simulink model "quadrotor_demo"  (Simulink 7.6)
settings: Solver=ode45  StartTime=0.0  StopTime=100  RelTol=1e-3
undefined symbols (not defined in the file): STARMAC, uav_utilities
libraries: simulink x9, aero_sim_lib x8
(part 1 of 2)
settings Model: Creator=Administrator  LastModifiedBy=jporter  SimulationMode=rapid-accelerator
settings OptimizationCC: InitFltsAndDblsToZero=on
settings DebuggingCC: SignalRangeChecking=warning  ParameterDowncastMsg=warning  ParameterOverflowMsg=warning
settings HardwareCC: ProdLargestAtomicInteger=Long  ProdLargestAtomicFloat=Float  ProdEndianess=LittleEndian  ProdHWDeviceType=ARM Compatible->ARM 7
settings SFSimCC: SimParseCustomCode=off

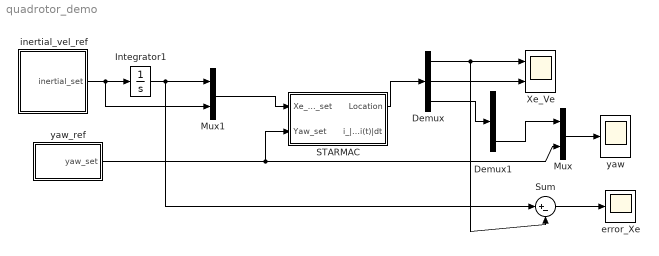
== system quadrotor_demo ==
  Demux : Demux  Outputs=[3,3,3]
  Demux1 : Demux  Outputs=3
  Integrator1 : Integrator
  Mux : Mux  Inputs=2
  Mux1 : Mux  Inputs=2
  STARMAC : Subsystem  AncestorBlock=uav_utilities/STARMAC  MinMaxOverflowLogging=MinMaxAndOverflow
  Sum : Sum  Inputs=|+-
  Xe_Ve : Scope  NumInputPorts=2
      settings: YMin=-500~-10  YMax=6500~110  SampleInput=on  SampleTime=100/5000
  error_Xe : Scope
      settings: YMin=-50  YMax=60  SaveName=error_data  Decimation=10  SampleInput=on  SampleTime=100/5000
  inertial_vel_ref : Subsystem
  yaw : Scope
      settings: YMin=-1  YMax=1  SaveName=ScopeData2  SampleInput=on  SampleTime=100/5000
  yaw_ref : Subsystem
  wires:
  inertial_vel_ref/1(inertial_set) -> Integrator1/1, Mux1/2
  yaw_ref/1(yaw_set) -> STARMAC/2(Yaw_set), Mux/2
  Sum/1 -> error_Xe/1
  STARMAC/1(Location) -> Demux/1
  Demux/1 -> Sum/2, Xe_Ve/1
  Demux/2 -> Xe_Ve/2
  Mux/1 -> yaw/1
  Demux/3 -> Demux1/1
  Demux1/3 -> Mux/1
  Integrator1/1 -> Mux1/1, Sum/1
  Mux1/1 -> STARMAC/1(Xe_Ve_set)

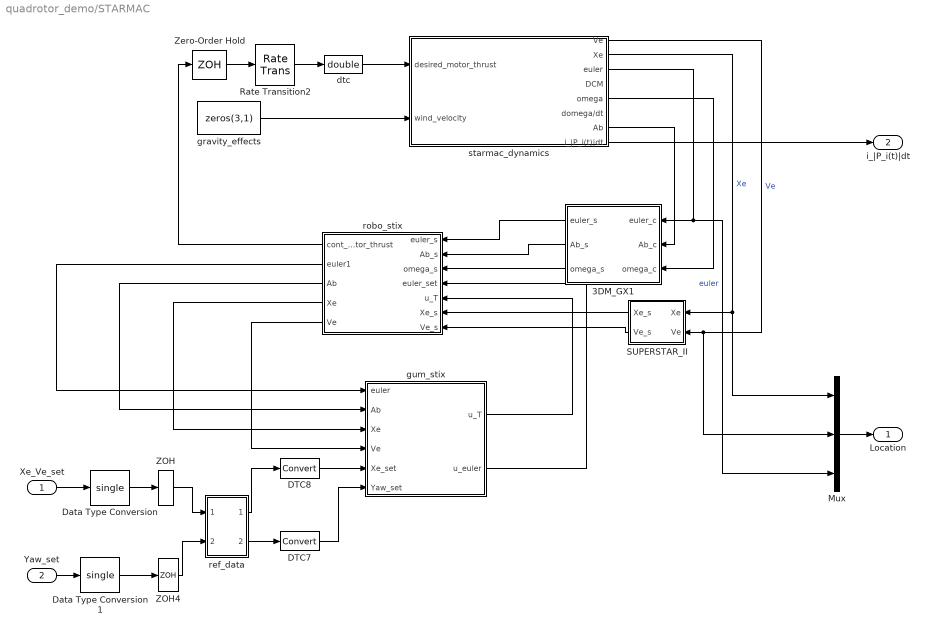
== system quadrotor_demo/STARMAC ==
  Xe_Ve_set : Inport  PortDimensions=[6]
  Yaw_set : Inport  Port=2  PortDimensions=[1]
  3DM_GX1 : Subsystem  mask{a_g_s=7000, g_max=5, g_g_s=8500, omega_max=300, Ts=.02}
      mask prompts: a_g_s "AccelGainScale:"; g_max "Max G (1 G = 9.81 m/s^2):"; g_g_s "GyroGainScale:"; omega_max "Mav Angular Velocity (deg/sec):"; Ts "Sample Rate (seconds):"
  DTC7 : DataTypeConversion
  DTC8 : DataTypeConversion
  Data Type Conversion : DataTypeConversion  OutDataTypeStr=single
  Data Type Conversion1 : DataTypeConversion  OutDataTypeStr=single
  Mux : Mux  Inputs=[3 3 3]
  Rate Transition2 : RateTransition
  SUPERSTAR_II : Subsystem  mask{Ts=.2}
      mask prompts: Ts "Sample Rate (seconds):"
  ZOH : ZeroOrderHold  SampleTime=.02
  ZOH4 : ZeroOrderHold  SampleTime=.02
  Zero-Order Hold : ZeroOrderHold  SampleTime=.02
  dtc : DataTypeConversion  OutDataTypeStr=double
  gravity_effects : Constant  Value=zeros(3,1)  OutDataTypeStr=double
  gum_stix : Subsystem
  ref_data : Subsystem
  robo_stix : Subsystem
  starmac_dynamics : Subsystem  AncestorBlock=aero_sim_lib/starmac_dynamics
  Location : Outport
  i_|P_i(t)|dt : Outport  Port=2
  wires:
  starmac_dynamics/8(i_|P_i(t)|dt) -> i_|P_i(t)|dt/1
  ref_data/2(Out2) -> DTC7/1
  Yaw_set/1 -> Data Type Conversion1/1
  Xe_Ve_set/1 -> Data Type Conversion/1
  Mux/1 -> Location/1
  robo_stix/1(cont_motor_thrust) -> Zero-Order Hold/1
  starmac_dynamics/3(euler) -> 3DM_GX1/1(euler_c), Mux/3  "euler"
  starmac_dynamics/7(Ab) -> 3DM_GX1/2(Ab_c)
  3DM_GX1/1(euler_s) -> robo_stix/1(euler_s)
  3DM_GX1/2(Ab_s) -> robo_stix/2(Ab_s)
  3DM_GX1/3(omega_s) -> robo_stix/3(omega_s)
  robo_stix/2(euler1) -> gum_stix/1(euler)
  SUPERSTAR_II/1(Xe_s) -> robo_stix/6(Xe_s)
  SUPERSTAR_II/2(Ve_s) -> robo_stix/7(Ve_s)
  starmac_dynamics/2(Xe) -> SUPERSTAR_II/1(Xe), Mux/1  "Xe"
  starmac_dynamics/1(Ve) -> SUPERSTAR_II/2(Ve), Mux/2  "Ve"
  gravity_effects/1 -> starmac_dynamics/2(wind_velocity)
  gum_stix/1(u_T) -> robo_stix/5(u_T)
  gum_stix/2(u_euler) -> robo_stix/4(euler_set)
  ref_data/1(Out1) -> DTC8/1
  dtc/1 -> starmac_dynamics/1(desired_motor_thrust)
  starmac_dynamics/5(omega) -> 3DM_GX1/3(omega_c)
  Zero-Order Hold/1 -> Rate Transition2/1
  Rate Transition2/1 -> dtc/1
  robo_stix/3(Ab) -> gum_stix/2(Ab)
  robo_stix/5(Ve) -> gum_stix/4(Ve)
  ZOH/1 -> ref_data/1(Xe_Ve_set)
  ZOH4/1 -> ref_data/2(yaw_set)
  Data Type Conversion/1 -> ZOH/1
  Data Type Conversion1/1 -> ZOH4/1
  DTC7/1 -> gum_stix/6(Yaw_set)
  DTC8/1 -> gum_stix/5(Xe_set)
  robo_stix/4(Xe) -> gum_stix/3(Xe)

== system quadrotor_demo/inertial_vel_ref ==
  Signal Generator : SignalGenerator  Amplitude=10*[1 -1 -.5]  Frequency=.1*.0625*ones(3,1)
  inertial_set : Outport
  wires:
  Signal Generator/1 -> inertial_set/1

== system quadrotor_demo/yaw_ref ==
  Signal Generator : SignalGenerator  Frequency=2*.0625*0.25
  yaw_set : Outport
  wires:
  Signal Generator/1 -> yaw_set/1

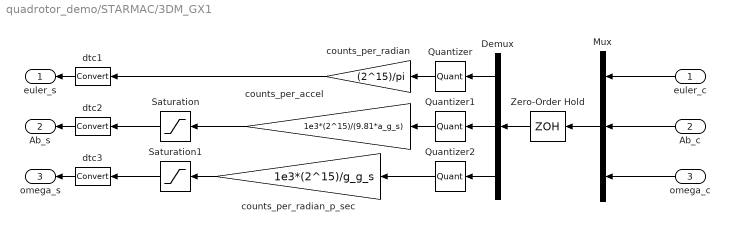
== system quadrotor_demo/STARMAC/3DM_GX1 ==
  euler_c : Inport
  Ab_c : Inport  Port=2
  omega_c : Inport  Port=3
  Demux : Demux  Outputs=[3 3 3]
  Mux : Mux  Inputs=[3 3 3]
  Quantizer : Quantizer  QuantizationInterval=pi/(2^15)*ones(3,1)
  Quantizer1 : Quantizer  QuantizationInterval=g_max*9.81/(2^15)*ones(3,1)
  Quantizer2 : Quantizer  QuantizationInterval=(pi*omega_max/180)/(2^15)*ones(3,1)
  Saturation : Saturate  UpperLimit=((2^15)-1)*ones(3,1)  LowerLimit=-(2^15)*ones(3,1)
  Saturation1 : Saturate  UpperLimit=((2^15)-1)*ones(3,1)  LowerLimit=-(2^15)*ones(3,1)
  Zero-Order Hold : ZeroOrderHold  SampleTime=Ts
  counts_per_accel : Gain  Gain=1e3*(2^15)/(9.81*a_g_s)  OutDataTypeStr=single
  counts_per_radian : Gain  Gain=(2^15)/pi  OutDataTypeStr=single
  counts_per_radian_p_sec : Gain  Gain=1e3*(2^15)/g_g_s  OutDataTypeStr=single
  dtc1 : DataTypeConversion
  dtc2 : DataTypeConversion
  dtc3 : DataTypeConversion
  euler_s : Outport
  Ab_s : Outport  Port=2
  omega_s : Outport  Port=3
  wires:
  Mux/1 -> Zero-Order Hold/1
  euler_c/1 -> Mux/1
  Ab_c/1 -> Mux/2
  omega_c/1 -> Mux/3
  Zero-Order Hold/1 -> Demux/1
  Demux/1 -> Quantizer/1
  Demux/2 -> Quantizer1/1
  Quantizer/1 -> counts_per_radian/1
  Quantizer1/1 -> counts_per_accel/1
  counts_per_accel/1 -> Saturation/1
  Demux/3 -> Quantizer2/1
  counts_per_radian_p_sec/1 -> Saturation1/1
  Quantizer2/1 -> counts_per_radian_p_sec/1
  Saturation/1 -> dtc2/1
  Saturation1/1 -> dtc3/1
  dtc1/1 -> euler_s/1
  dtc2/1 -> Ab_s/1
  dtc3/1 -> omega_s/1
  counts_per_radian/1 -> dtc1/1

== system quadrotor_demo/STARMAC/SUPERSTAR_II ==
  Xe : Inport
  Ve : Inport  Port=2
  Demux : Demux  Outputs=[3 3]
  Mux : Mux  Inputs=[3 3]
  Rate Transition : RateTransition
  ZOH : ZeroOrderHold  SampleTime=Ts
  dtc1 : DataTypeConversion
  dtc2 : DataTypeConversion
  Xe_s : Outport
  Ve_s : Outport  Port=2
  wires:
  ZOH/1 -> Rate Transition/1
  Ve/1 -> Mux/2
  Xe/1 -> Mux/1
  Mux/1 -> ZOH/1
  Demux/1 -> dtc1/1
  Demux/2 -> dtc2/1
  dtc1/1 -> Xe_s/1
  dtc2/1 -> Ve_s/1
  Rate Transition/1 -> Demux/1

== system quadrotor_demo/STARMAC/gum_stix ==
  euler : Inport  OutMin=-pi  OutMax=pi  OutDataTypeStr=fixdt(1,32,28)  PortDimensions=[3]
  Ab : Inport  Port=2  OutMin=-200  OutMax=200  OutDataTypeStr=fixdt(1,32,23)  PortDimensions=[3]
  Xe : Inport  Port=3  OutMin=-2000  OutMax=2000  OutDataTypeStr=fixdt(1,32,20)  PortDimensions=[3]
  Ve : Inport  Port=4  OutMin=-200  OutMax=200  OutDataTypeStr=fixdt(1,32,23)  PortDimensions=[3]
  Xe_set : Inport  Port=5  OutMin=-2000  OutMax=2000  OutDataTypeStr=fixdt(1,32,20)  PortDimensions=[3]
  Yaw_set : Inport  Port=6  OutMin=-pi  OutMax=pi  OutDataTypeStr=fixdt(1,32,29)  PortDimensions=[1]
  DTC : DataTypeConversion
  Demux : Demux  Outputs=3
  body_to_inertial : Subsystem
  inertial_pos_controller : Subsystem
  rate_limiter : Subsystem  mask{wn=2*pi, zeta=0.9, Vmax=2, T=0.02, Hzn1=0, Hzd1=0}
      mask prompts: wn "omega_n"; Vmax "Max velocity"; T "Sample time"; Hzn1 "Filter numerator"; Hzd1 "Filter denominator"
      mask init:
      | Hs=tf([wn^2],[1,2*zeta*wn,wn^2]);
      | Hz=ipesh_transform(Hs,T);
      | Hzn1 = Hz.num{1};
      | %Hzn1 = [0.002488 0.009405 0.002222];
      | Hzd1 = Hz.den{1};
      | %Hzd1 = [1.0000 -1.7834 0.7976];
  sensor_fusion : Subsystem
  u_T : Outport  OutMin=0  OutMax=100  PortDimensions=[1]
  u_euler : Outport  Port=2  OutMin=-pi  OutMax=pi  PortDimensions=[3]
  wires:
  Xe_set/1 -> rate_limiter/1(Xe_set)
  inertial_pos_controller/1(u_T) -> u_T/1
  inertial_pos_controller/2(u_euler) -> u_euler/1
  euler/1 -> body_to_inertial/1(euler), Demux/1
  Ab/1 -> DTC/1
  sensor_fusion/1(Xe) -> inertial_pos_controller/2(Xe)
  sensor_fusion/2(Ve) -> inertial_pos_controller/3(Ve)
  body_to_inertial/1(Xe) -> sensor_fusion/1(Xe_f)
  body_to_inertial/2(Ve) -> sensor_fusion/2(Ve_f)
  Xe/1 -> sensor_fusion/3(Xe_s)
  Ve/1 -> sensor_fusion/4(Ve_s)
  rate_limiter/1(Xr_set) -> inertial_pos_controller/1(Xe_set)
  Demux/3 -> inertial_pos_controller/4(Yaw_actual)
  Yaw_set/1 -> inertial_pos_controller/5(Yaw_set)
  DTC/1 -> body_to_inertial/2(Ab)

== system quadrotor_demo/STARMAC/ref_data ==
  Xe_Ve_set : Inport  PortDimensions=[6]
  yaw_set : Inport  Port=2  PortDimensions=[1]
  Data Type Conversion : DataTypeConversion
  Data Type Conversion1 : DataTypeConversion
  Demux : Demux  Outputs=[3,3]
  Terminator : Terminator
  Out1 : Outport
  Out2 : Outport  Port=2
  wires:
  Demux/2 -> Terminator/1
  Demux/1 -> Data Type Conversion/1
  Data Type Conversion/1 -> Out1/1
  Xe_Ve_set/1 -> Demux/1
  Data Type Conversion1/1 -> Out2/1
  yaw_set/1 -> Data Type Conversion1/1

== system quadrotor_demo/STARMAC/robo_stix ==
  euler_s : Inport  OutMin=-(2^15)  OutMax=2^15  OutDataTypeStr=fixdt(1,32,15)  PortDimensions=[3]
  Ab_s : Inport  Port=2  OutMin=-(2^15)  OutMax=2^15  OutDataTypeStr=fixdt(1,32,15)  PortDimensions=[3]
  omega_s : Inport  Port=3  OutMin=-(2^15)  OutMax=2^15  OutDataTypeStr=fixdt(1,32,15)  PortDimensions=[3]
  euler_set : Inport  Port=4  OutMin=-pi  OutMax=pi  OutDataTypeStr=fixdt(1,32,29)  PortDimensions=[3]
  u_T : Inport  Port=5  OutMin=0  OutMax=100  OutDataTypeStr=fixdt(1,32,24)  PortDimensions=[1]
  Xe_s : Inport  Port=6  OutMin=-2000  OutMax=2000  OutDataTypeStr=fixdt(1,32,20)  PortDimensions=[3]
  Ve_s : Inport  Port=7  OutMin=-200  OutMax=200  OutDataTypeStr=fixdt(1,32,23)  PortDimensions=[3]
  inner_loop : Subsystem
  sensor_convert : Subsystem  mask{a_g_s=7000, g_g_s=8500}
      mask prompts: a_g_s "AccelGainScale[a_g_s]:"; g_g_s "GyroGainScale[g_g_s]:"
  cont_motor_thrust : Outport
  euler1 : Outport  Port=2
  Ab : Outport  Port=3
  Xe : Outport  Port=4
  Ve : Outport  Port=5
  wires:
  euler_s/1 -> sensor_convert/1(euler_s)
  Ab_s/1 -> sensor_convert/2(Ab_s)
  omega_s/1 -> sensor_convert/3(omega_s)
  sensor_convert/1(euler_il) -> inner_loop/2(euler)
  euler_set/1 -> inner_loop/1(euler_s)
  sensor_convert/3(omega) -> inner_loop/3(omega)
  u_T/1 -> inner_loop/4(u_T)
  sensor_convert/2(Ab) -> Ab/1
  inner_loop/1(thrust) -> cont_motor_thrust/1
  Xe_s/1 -> sensor_convert/4(Xe_s)
  Ve_s/1 -> sensor_convert/5(Ve_s)
  sensor_convert/4(Xe) -> Xe/1
  sensor_convert/5(Ve) -> Ve/1
  sensor_convert/6(euler_ol) -> euler1/1

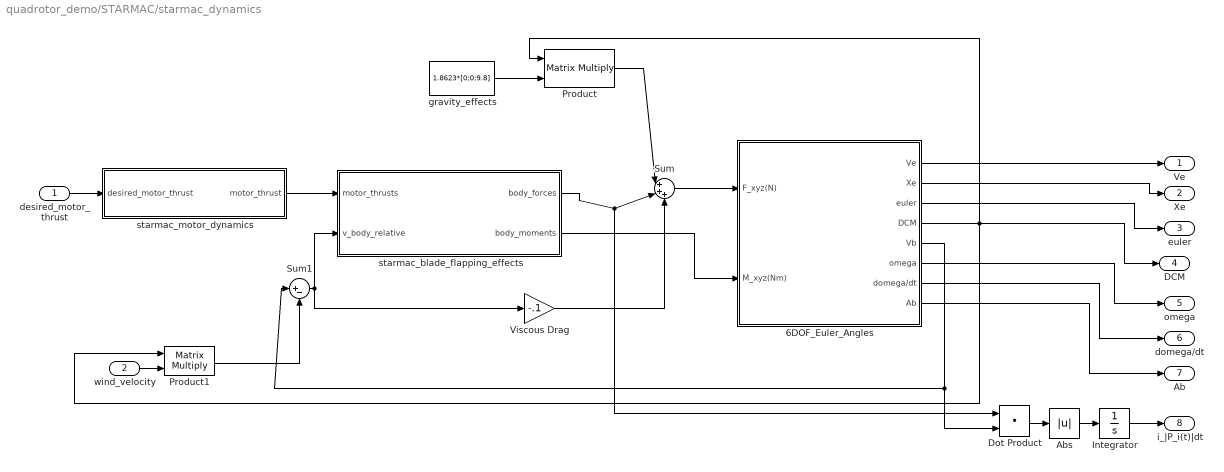
== system quadrotor_demo/STARMAC/starmac_dynamics ==
  desired_motor_thrust : Inport
  wind_velocity : Inport  Port=2
  6DOF_Euler_Angles : Subsystem  AncestorBlock=aero_sim_lib/6DOF (Euler Angles)_CMU  mask{XYZe_0=[0.1;0.2;0], Vb_0=[0;0;0], euler_0=[0;0;0], omega_0=[0;0;0], M=1.8623, I=diag([0.02759 0.02771 0.04806])}
      mask prompts: XYZe_0 "Initial position in inertial axes [Xe,Ye,Ze]:"; Vb_0 "Initial velocity in body axes [U,v,w]:"; euler_0 "Initial Euler orientation [roll, pitch, yaw]=[phi,theta,psi]:"; omega_0 "Initial body rotation rates [p,q,r]=omega:"; M "Initial mass:"; I "Inertial:"
  Abs : Abs
  Dot Product : DotProduct  InputSameDT=on  OutDataTypeStr=Inherit: Inherit via internal rule
  Integrator : Integrator
  Product : Product  Multiplication=Matrix(*)  RndMeth=Zero
  Product1 : Product  Multiplication=Matrix(*)  RndMeth=Zero
  Sum : Sum  Inputs=|+++
  Sum1 : Sum  Inputs=|+-
  Viscous Drag : Gain  Gain=-.1  OutDataTypeStr=single
  gravity_effects : Constant  Value=1.8623*[0;0;9.8]
  starmac_blade_flapping_effects : Subsystem  AncestorBlock=aero_sim_lib/starmac_blade_flapping_effects
  starmac_motor_dynamics : Subsystem  AncestorBlock=aero_sim_lib/starmac_motor_dynamics  mask{tau_motor=.1, T_nom=1.8263*9.8/4, thrust_max=9.8, thrust_min=0, motor_lag_enable=on, motor_variance=.01*(.05*9.8/4)^2, Ts=1/76}
      mask prompts: tau_motor "tau_motor (seconds):"; T_nom "nominal thrust (N):"; thrust_max "maximum thrust (N):"; thrust_min "minimum thrust (N):"; motor_lag_enable "Motor Lag Enabled:"; motor_variance "Motor Variance [motor_variance]:"; Ts "Motor Update Rate (seconds):"
  Ve : Outport
  Xe : Outport  Port=2
  euler : Outport  Port=3
  DCM : Outport  Port=4
  omega : Outport  Port=5
  domega/dt : Outport  Port=6
  Ab : Outport  Port=7
  i_|P_i(t)|dt : Outport  Port=8
  wires:
  wind_velocity/1 -> Product1/2
  desired_motor_thrust/1 -> starmac_motor_dynamics/1(desired_motor_thrust)
  starmac_blade_flapping_effects/1(body_forces) -> Sum/2, Dot Product/1
  starmac_blade_flapping_effects/2(body_moments) -> 6DOF_Euler_Angles/2(M_xyz(Nm))
  Viscous Drag/1 -> Sum/3
  6DOF_Euler_Angles/5(Vb) -> Sum1/1, Dot Product/2
  Product1/1 -> Sum1/2
  Sum1/1 -> Viscous Drag/1, starmac_blade_flapping_effects/2(v_body_relative)
  gravity_effects/1 -> Product/2
  6DOF_Euler_Angles/4(DCM) -> Product1/1, Product/1, DCM/1
  Sum/1 -> 6DOF_Euler_Angles/1(F_xyz(N))
  Product/1 -> Sum/1
  starmac_motor_dynamics/1(motor_thrust) -> starmac_blade_flapping_effects/1(motor_thrusts)
  6DOF_Euler_Angles/1(Ve) -> Ve/1
  6DOF_Euler_Angles/2(Xe) -> Xe/1
  6DOF_Euler_Angles/3(euler) -> euler/1
  6DOF_Euler_Angles/6(omega) -> omega/1
  6DOF_Euler_Angles/7(domega/dt) -> domega/dt/1
  6DOF_Euler_Angles/8(Ab) -> Ab/1
  Integrator/1 -> i_|P_i(t)|dt/1
  Dot Product/1 -> Abs/1
  Abs/1 -> Integrator/1

== system quadrotor_demo/STARMAC/gum_stix/body_to_inertial ==
  euler : Inport
  Ab : Inport  Port=2
  Ab_to_Ae_subsys : Subsystem
  inertial_vel_and pos_est : Subsystem  mask{Ts=.02}
      mask prompts: Ts "Sample Time [Ts] (seconds):"
  Xe : Outport
  Ve : Outport  Port=2
  wires:
  euler/1 -> Ab_to_Ae_subsys/1(In1)
  Ab/1 -> Ab_to_Ae_subsys/2(In2)
  inertial_vel_and pos_est/1(Vb) -> Ve/1
  inertial_vel_and pos_est/2(Xb) -> Xe/1
  Ab_to_Ae_subsys/1(Out1) -> inertial_vel_and pos_est/1(Ab)

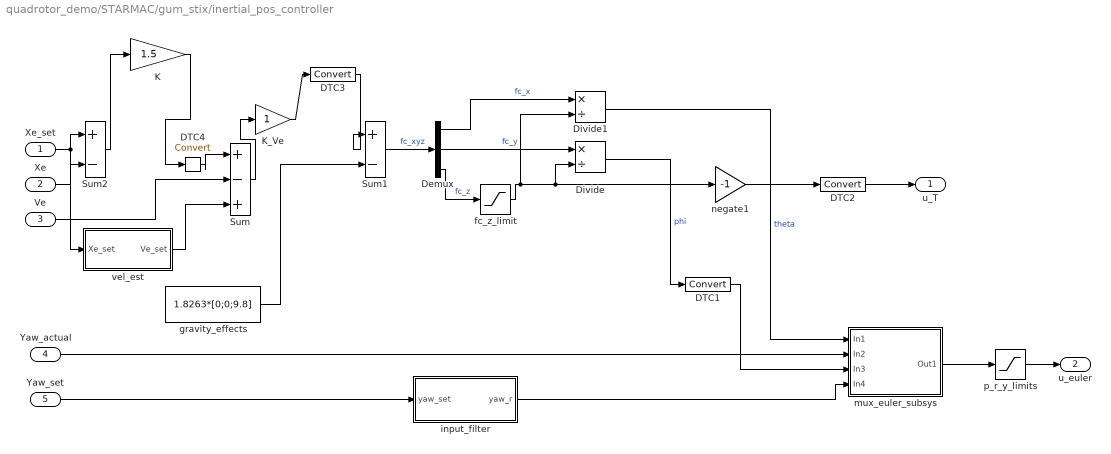
== system quadrotor_demo/STARMAC/gum_stix/inertial_pos_controller ==
  Xe_set : Inport
  Xe : Inport  Port=2
  Ve : Inport  Port=3
  Yaw_actual : Inport  Port=4
  Yaw_set : Inport  Port=5
  DTC{1..4} (4 alike) : DataTypeConversion
  Demux : Demux  Outputs=3
  Divide : Product  Inputs=*/  OutDataTypeStr=fixdt(1,32,23)
  Divide1 : Product  Inputs=*/  OutDataTypeStr=fixdt(1,32,23)
  K : Gain  Gain=1.5  OutDataTypeStr=fixdt(1,32,19)
  K_Ve : Gain  OutDataTypeStr=fixdt(1,32,19)
  Sum : Sum  Inputs=|+-+  OutDataTypeStr=fixdt(1,32,19)
  Sum1 : Sum  Inputs=|+-  OutDataTypeStr=fixdt(1,32,19)
  Sum2 : Sum  Inputs=|+-  OutDataTypeStr=fixdt(1,32,19)
  fc_z_limit : Saturate  UpperLimit=-(1/8)*9.81  LowerLimit=-4*9.81  OutDataTypeStr=fixdt(1,32,25)
  gravity_effects : Constant  Value=1.8263*[0;0;9.8]  OutDataTypeStr=fixdt(1,32,26)
  input_filter : Subsystem  mask{wn=1, zeta=0.9, T=0.01}
      mask prompts: wn "omega_n"; T "Sample time"
      mask init:
      | Hs=tf([wn^2],[1,2*zeta*wn,wn^2]);
      | Hz=ipesh_transform(Hs,T);
  mux_euler_subsys : Subsystem
  negate1 : Gain  Gain=-1  OutDataTypeStr=fixdt(1,32,25)
  p_r_y_limits : Saturate  UpperLimit=[pi/4,pi/4,inf]  LowerLimit=-[pi/4,pi/4,inf]  OutDataTypeStr=fixdt(1,32,29)
  vel_est : Subsystem  mask{tau_f=.01/pi, T=.01}
      mask prompts: T "sample rate"
      mask init:
      | %b=1/tau_f;
      | %num1=(1-exp(-b*T));
      | %num2=-num1;
      | %den1=1;
      | %den2=-exp(-b*T);
      | %num=(1/T)*[num1 num2];
      | %den=[den1 den2];
      | %vel_est_a_1=single(-den(2)/den(1))
      | %vel_est_b_1=single(num(2)/den(1))
      | %vel_est_b_2=single(num(1)/den(1))
      | Hs=tf([1 0],[T/pi 1]);
      | Hz=ipesh_transform(Hs,T);
      | %Hz=tf(num,den,T);
      | %bode(Hz);
      | %hold on;
      | %bode(tf([1 0],[tau_f 1]));
  u_T : Outport
  u_euler : Outport  Port=2
  wires:
  fc_z_limit/1 -> Divide1/2, Divide/2, negate1/1
  Xe_set/1 -> Sum2/1, vel_est/1(Xe_set)
  negate1/1 -> DTC2/1
  p_r_y_limits/1 -> u_euler/1
  Demux/1 -> Divide1/1  "fc_x"
  Demux/3 -> fc_z_limit/1  "fc_z"
  Sum1/1 -> Demux/1  "fc_xyz"
  gravity_effects/1 -> Sum1/2
  Sum/1 -> K_Ve/1
  Xe/1 -> Sum2/2
  Sum2/1 -> K/1
  K/1 -> DTC4/1
  Demux/2 -> Divide/1  "fc_y"
  K_Ve/1 -> DTC3/1
  Ve/1 -> Sum/2
  vel_est/1(Ve_set) -> Sum/3
  Yaw_set/1 -> input_filter/1(yaw_set)
  Divide1/1 -> mux_euler_subsys/1(In1)  "theta"
  Divide/1 -> DTC1/1  "phi"
  Yaw_actual/1 -> mux_euler_subsys/2(In2)
  input_filter/1(yaw_r) -> mux_euler_subsys/4(In4)
  mux_euler_subsys/1(Out1) -> p_r_y_limits/1
  DTC1/1 -> mux_euler_subsys/3(In3)
  DTC2/1 -> u_T/1
  DTC3/1 -> Sum1/1
  DTC4/1 -> Sum/1

== system quadrotor_demo/STARMAC/gum_stix/rate_limiter ==
  Xe_set : Inport
  Constant : Constant  Value=T  OutDataTypeStr=fixdt(1,32,31)
  Constant1 : Constant  Value=Vmax  OutDataTypeStr=fixdt(1,32,10)
  DTC : DataTypeConversion
  DTC1 : DataTypeConversion
  DTC2 : DataTypeConversion
  Demux : Demux  Outputs=3
  Discrete Transfer Fcn : DiscreteTransferFcn  Numerator=Hzn1  Denominator=Hzd1  SampleTime=-1
  Discrete Transfer Fcn1 : DiscreteTransferFcn  Numerator=Hzn1  Denominator=Hzd1  SampleTime=-1
  Discrete Transfer Fcn2 : DiscreteTransferFcn  Numerator=Hzn1  Denominator=Hzd1  SampleTime=-1
  Mux : Mux  Inputs=3
  Unit Delay : UnitDelay  SampleTime=-1
  limit_rate_subsys : Subsystem
  Xr_set : Outport
  wires:
  Xe_set/1 -> Demux/1
  Mux/1 -> limit_rate_subsys/2(Xd_prev)
  limit_rate_subsys/1(Xr) -> Xr_set/1, Unit Delay/1
  Constant/1 -> limit_rate_subsys/3(Tsamp)
  Constant1/1 -> limit_rate_subsys/4(Vmax)
  Demux/1 -> Discrete Transfer Fcn/1
  Discrete Transfer Fcn/1 -> DTC/1
  Demux/2 -> Discrete Transfer Fcn1/1
  Discrete Transfer Fcn1/1 -> DTC1/1
  Demux/3 -> Discrete Transfer Fcn2/1
  Discrete Transfer Fcn2/1 -> DTC2/1
  DTC/1 -> Mux/1
  DTC1/1 -> Mux/2
  DTC2/1 -> Mux/3
  Unit Delay/1 -> limit_rate_subsys/1(Xd)

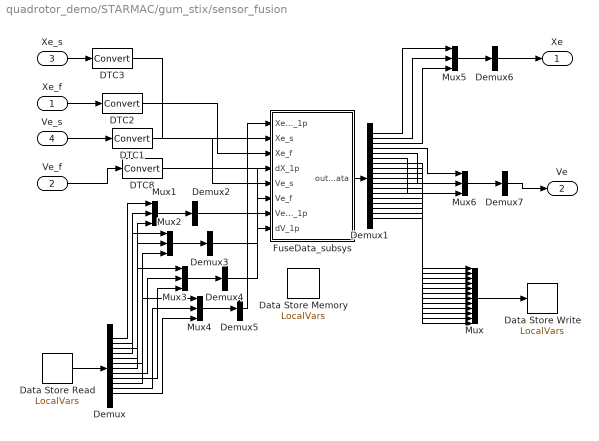
== system quadrotor_demo/STARMAC/gum_stix/sensor_fusion ==
  Xe_f : Inport
  Ve_f : Inport  Port=2
  Xe_s : Inport  Port=3
  Ve_s : Inport  Port=4
  DTC{1..3,8} (4 alike) : DataTypeConversion  LockScale=on
  Data Store Memory : DataStoreMemory  DataStoreName=LocalVars  ReadBeforeWriteMsg=warning  WriteAfterWriteMsg=warning  WriteAfterReadMsg=warning  InitialValue=zeros(12,1)
  Data Store Read : DataStoreRead  DataStoreName=LocalVars
  Data Store Write : DataStoreWrite  DataStoreName=LocalVars
  Demux : Demux  Outputs=12
  Demux1 : Demux  Outputs=18
  Demux{2..7} (6 alike) : Demux  Outputs=1
  FuseData_subsys : Subsystem
  Mux : Mux  Inputs=12
  Mux{1..6} (6 alike) : Mux  Inputs=3
  Xe : Outport
  Ve : Outport  Port=2
  wires:
  Xe_s/1 -> DTC3/1
  Xe_f/1 -> DTC2/1
  Ve_s/1 -> DTC1/1
  Ve_f/1 -> DTC8/1
  Data Store Read/1 -> Demux/1
  Mux/1 -> Data Store Write/1
  Demux/1 -> Mux1/1
  Demux/2 -> Mux1/2
  Demux/3 -> Mux1/3
  Mux1/1 -> Demux2/1
  Demux2/1 -> FuseData_subsys/8(dV_1p)
  Demux/4 -> Mux2/1
  Demux/5 -> Mux2/2
  Demux/6 -> Mux2/3
  Mux2/1 -> Demux3/1
  Demux3/1 -> FuseData_subsys/4(dX_1p)
  Demux/7 -> Mux3/1
  Demux/8 -> Mux3/2
  Demux/9 -> Mux3/3
  Mux3/1 -> Demux4/1
  Demux4/1 -> FuseData_subsys/7(Ve_sh_1p)
  Demux/10 -> Mux4/1
  Demux/11 -> Mux4/2
  Demux/12 -> Mux4/3
  Mux4/1 -> Demux5/1
  Demux5/1 -> FuseData_subsys/1(Xe_sh_1p)
  Mux5/1 -> Demux6/1
  Mux6/1 -> Demux7/1
  Demux1/1 -> Mux5/1
  Demux1/2 -> Mux5/2
  Demux1/3 -> Mux5/3
  Demux1/4 -> Mux6/1
  Demux1/5 -> Mux6/2
  Demux1/6 -> Mux6/3
  Demux1/7 -> Mux/1
  Demux1/8 -> Mux/2
  Demux1/9 -> Mux/3
  Demux1/10 -> Mux/4
  Demux1/11 -> Mux/5
  Demux1/12 -> Mux/6
  Demux1/13 -> Mux/7
  Demux1/14 -> Mux/8
  Demux1/15 -> Mux/9
  Demux1/16 -> Mux/10
  Demux1/17 -> Mux/11
  Demux1/18 -> Mux/12
  Demux6/1 -> Xe/1
  Demux7/1 -> Ve/1
  DTC8/1 -> FuseData_subsys/6(Ve_f)
  DTC1/1 -> FuseData_subsys/5(Ve_s)
  DTC2/1 -> FuseData_subsys/3(Xe_f)
  DTC3/1 -> FuseData_subsys/2(Xe_s)
  FuseData_subsys/1(out_data) -> Demux1/1

== system quadrotor_demo/STARMAC/robo_stix/inner_loop ==
  euler_s : Inport  PortDimensions=[3]
  euler : Inport  Port=2  OutDataTypeStr=fixdt(1,32,31)  PortDimensions=[3]
  omega : Inport  Port=3  OutDataTypeStr=fixdt(1,32,33)  PortDimensions=[3]
  u_T : Inport  Port=4  OutDataTypeStr=fixdt(1,32,24)  PortDimensions=[1]
  euler_controller : Subsystem  mask{K=1, K_e=7.5/.65, K_o=.5}
      mask prompts: K "Loop Gain [K]:"; K_e "Euler Gain [K_e]:"; K_o "Omega Gain [K_o]:"
  lead_motor : Subsystem  mask{tau_motor=0.1, t_s=0.02, Hzn1=0, Hzd1=0}
      mask prompts: Hzn1 "Filter numerator"; Hzd1 "Filter denominator"
      mask init:
      | Hs=tf([tau_motor 1],[t_s/pi 1]);
      | Hz=ipesh_transform(Hs,t_s);
      | Hzn1 = Hz.num{1};
      | %Hzn1 = [5.4794 -4.52326];
      | Hzd1 = Hz.den{1};
      | %Hzd1 = [1.0000 -0.04321];
      | 
      | %a=1/tau_motor;
      | %b=pi/t_s;
      | %T=t_s;
      | %num1=b*(1-exp(-b*T))+a*(b*T-1+exp(-b*T));
      | %num2=-b*(1-exp(-b*T))+a*(1-exp(-b*T)-b*T*exp(-b*T));
      | %den1=a*b;
      | %den2=-a*b*exp(-b*T);
      | %num=[num1 num2];
      | %den=[den1 den2];
      | %Hz=tf(num,den,T);
      | %[y,t]=step(Hz);
      | %k_ss=(1/y(length(y)));
      | %num=k_ss*num;
      | %lead_a_1=single(-den(2)/den(1))
      | %lead_b_1=single(num(2)/den(1))
      | %lead_b_2=single(num(1)/den(1))
      | %Hz=k_ss*Hz
      | %bode(Hz);
  thrust_limit : Saturate  UpperLimit=10*ones(4,1)  LowerLimit=0*ones(4,1)  OutDataTypeStr=fixdt(1,32,27)
  u_T_u_torque_motor_thrust : Subsystem  mask{dx=0.1, K_torque=.47}
      mask prompts: dx "X distance of motor from CG [dx](meters):"; K_torque "Ktorque [K_torque]:"
      mask init:
      | M=[0 -dx 0 dx;
      |    dx 0 -dx 0;
      |    -K_torque K_torque -K_torque K_torque;
      |    1 1 1 1];
      | Mi=single(inv(M));
  thrust : Outport  OutDataTypeStr=fixdt(1,32,27)  PortDimensions=[4]
  wires:
  euler_controller/1(u_torque) -> u_T_u_torque_motor_thrust/1(u_torque)
  u_T_u_torque_motor_thrust/1(cont_motor_thrust) -> lead_motor/1(thrust_in)
  lead_motor/1(thrust_out) -> thrust_limit/1
  euler/1 -> euler_controller/2(euler)
  euler_s/1 -> euler_controller/1(euler_set)
  thrust_limit/1 -> thrust/1
  omega/1 -> euler_controller/3(omega)
  u_T/1 -> u_T_u_torque_motor_thrust/2(u_T)

== system quadrotor_demo/STARMAC/robo_stix/sensor_convert ==
  euler_s : Inport  PortDimensions=[3]
  Ab_s : Inport  Port=2  PortDimensions=[3]
  omega_s : Inport  Port=3  PortDimensions=[3]
  Xe_s : Inport  Port=4  PortDimensions=[3]
  Ve_s : Inport  Port=5  PortDimensions=[3]
  Data Type Conversion{,1..3} (4 alike) : DataTypeConversion
  accel_per_count : Gain  Gain=(9.81*a_g_s)/(1e3*32768)
  radian_p_sec_per_count : Gain  Gain=g_g_s/(1e3*32768)
  radian_per_count : Gain  Gain=pi/32768
  euler_il : Outport
  Ab : Outport  Port=2
  omega : Outport  Port=3
  Xe : Outport  Port=4
  Ve : Outport  Port=5
  euler_ol : Outport  Port=6
  wires:
  euler_s/1 -> radian_per_count/1
  radian_per_count/1 -> Data Type Conversion2/1, Data Type Conversion3/1
  Ab_s/1 -> accel_per_count/1
  accel_per_count/1 -> Data Type Conversion1/1
  omega_s/1 -> radian_p_sec_per_count/1
  radian_p_sec_per_count/1 -> Data Type Conversion/1
  Xe_s/1 -> Xe/1
  Ve_s/1 -> Ve/1
  Data Type Conversion/1 -> omega/1
  Data Type Conversion1/1 -> Ab/1
  Data Type Conversion2/1 -> euler_il/1
  Data Type Conversion3/1 -> euler_ol/1

== system quadrotor_demo/STARMAC/starmac_dynamics/6DOF_Euler_Angles ==
  note: This subsystem models a 6 degree of freedom (6DOF) system in Euler angles.
      | A Direct Cosine Matrix (DCM) is produced to allow for easy transformations to
      | and from the reference frame of the body.  Enter appropriate Parameters in the dialog menu.
      | Follows Euler Angle Sequence (1,2,3), see Section 5.6, Representing Attitude: Euler Angles, Unit
      | Quaternions, and Rotation by James Diebel.  Interface matches that from the Aerospace Toolbox
      | for non variable mass (6DoF EoM (Body Axis) for Euler Angles).
      |
      | J. Kapinski
      | Carnegia Mellon University
      | 7/2007
      | Revised:
      | Nicholas Kottenstette, ISIS, 8/2008
  note: 6 DOF System Model
  F_xyz(N) : Inport
  M_xyz(Nm) : Inport  Port=2  PortDimensions=3
  body_euler_to_earth : aero_sim_lib/body_euler_to_earth  SystemSampleTime=-1  XYZe_0=XYZe_0
  continuous_body_dynamics : aero_sim_lib/continuous_body_dynamics  SystemSampleTime=-1  M=M  Vb_0=Vb_0
  continuous_inertia_body_dynamics : aero_sim_lib/continuous_inertia_body_dynamics  SystemSampleTime=-1  I=I  omega_0=omega_0
  omega_to_euler : aero_sim_lib/omega_to_euler  SystemSampleTime=-1  euler_0=euler_0
  Ve : Outport
  Xe : Outport  Port=2
  euler : Outport  Port=3
  DCM : Outport  Port=4
  Vb : Outport  Port=5
  omega : Outport  Port=6
  domega/dt : Outport  Port=7
  Ab : Outport  Port=8
  wires:
  body_euler_to_earth/3 -> Xe/1
  body_euler_to_earth/2 -> DCM/1
  body_euler_to_earth/1 -> Ve/1
  omega_to_euler/1 -> body_euler_to_earth/1, euler/1
  continuous_inertia_body_dynamics/2 -> domega/dt/1
  continuous_body_dynamics/2 -> Ab/1
  continuous_body_dynamics/1 -> body_euler_to_earth/2, Vb/1
  continuous_inertia_body_dynamics/1 -> omega_to_euler/1, continuous_body_dynamics/2, omega/1
  F_xyz(N)/1 -> continuous_body_dynamics/1
  M_xyz(Nm)/1 -> continuous_inertia_body_dynamics/1

== system quadrotor_demo/STARMAC/starmac_dynamics/starmac_blade_flapping_effects ==
  motor_thrusts : Inport
  v_body_relative : Inport  Port=2
  Pick First 2 Elements : Constant  Value=[1 0 0; 0 1 0; 0 0 0]
  Product : Product  RndMeth=Zero
  Product2 : Product  Multiplication=Matrix(*)  RndMeth=Zero
  Product4 : Product  RndMeth=Zero
  Sum : Sum  Inputs=|++
  Sum of Elements : Sum  Inputs=+
  starmac_body_moments : Subsystem  AncestorBlock=aero_sim_lib/starmac_body_moments  mask{dx=.3048, dz=.07, K_torque=.47}
  starmac_flapping_dynamics : Subsystem  AncestorBlock=aero_sim_lib/starmac_flapping_dynamics  mask{K_a1s=.009, K_beta=.23}
  starmac_vertical_effect_dynamics : Subsystem  AncestorBlock=aero_sim_lib/starmac_vertical_effect_dynamics  mask{tau_motor=0.1, R=0.127, Alpha=(pi/180)*[-85:5:85], Vinf=[0:0.5:6], Thrust=9.8*[0.3:0.02:0.8]}
      mask prompts: tau_motor "motor time constant (s)"; R "radius of propeller (m)"; Alpha "Alpha (radians)"; Vinf "Vinf (radians)"; Thrust "Propeller Thrust (N)"
      mask init:
      | rho = 1.2;
      | A = pi*R^2;
      | Vh = sqrt(Thrust/(2*rho*A));
      | for i = 1:length(Vh)
      |     for j = 1:length(Vinf)
      |         for k = 1:length(Alpha)
      |             Vi(k,j,i) = find_vi(Vh(i),Vinf(j),Alpha(k));
      |             ToverTh(k,j,i) = min(10,max(0.1,Vh(i)/(Vi(k,j,i)+Vinf(j)*sin(Alpha(k)))));
      |         end
      |     end
      | end
  body_forces : Outport
  body_moments : Outport  Port=2
  wires:
  starmac_flapping_dynamics/2(rotor_blade_moments) -> Sum/2
  Sum/1 -> body_moments/1
  starmac_body_moments/1(Body Moments) -> Sum/1
  starmac_flapping_dynamics/1(thrust_vector) -> Product4/2, starmac_body_moments/2(Thrust Vector)
  Product4/1 -> body_forces/1
  Sum of Elements/1 -> Product4/1
  Product2/1 -> starmac_flapping_dynamics/1(Vb2_hat)
  v_body_relative/1 -> Product2/2, starmac_vertical_effect_dynamics/2(v_body_relative)
  Pick First 2 Elements/1 -> Product2/1
  motor_thrusts/1 -> Product/1, starmac_vertical_effect_dynamics/1(motor_thrusts)
  starmac_vertical_effect_dynamics/1(thrust_multiplier) -> Product/2
  Product/1 -> Sum of Elements/1, starmac_body_moments/1(Thrust Magnitudes)

== system quadrotor_demo/STARMAC/starmac_dynamics/starmac_motor_dynamics ==
  desired_motor_thrust : Inport
  Band-Limited White Noise : simulink/Sources/Band-Limited White Noise  SystemSampleTime=-1  Cov=Ts*motor_variance*ones(4,1)  Ts=Ts  seed=22341+[0 1 2 3]'
  Constant : Constant  Value=motor_lag_enable
  Saturation : Saturate  UpperLimit=thrust_max*ones(4,1)  LowerLimit=thrust_min*ones(4,1)
  State-Space : StateSpace  A=-(1/tau_motor)*eye(4)  B=(1/tau_motor)*eye(4)  C=eye(4)  D=zeros(4,4)  X0=T_nom*ones(4,1)
  Sum : Sum  Inputs=|++
  Switch : Switch  Criteria=u2 > Threshold
  motor_thrust : Outport
  wires:
  desired_motor_thrust/1 -> State-Space/1, Switch/3
  Sum/1 -> motor_thrust/1
  Saturation/1 -> Sum/1
  Band-Limited White Noise/1 -> Sum/2
  State-Space/1 -> Switch/1
  Switch/1 -> Saturation/1
  Constant/1 -> Switch/2

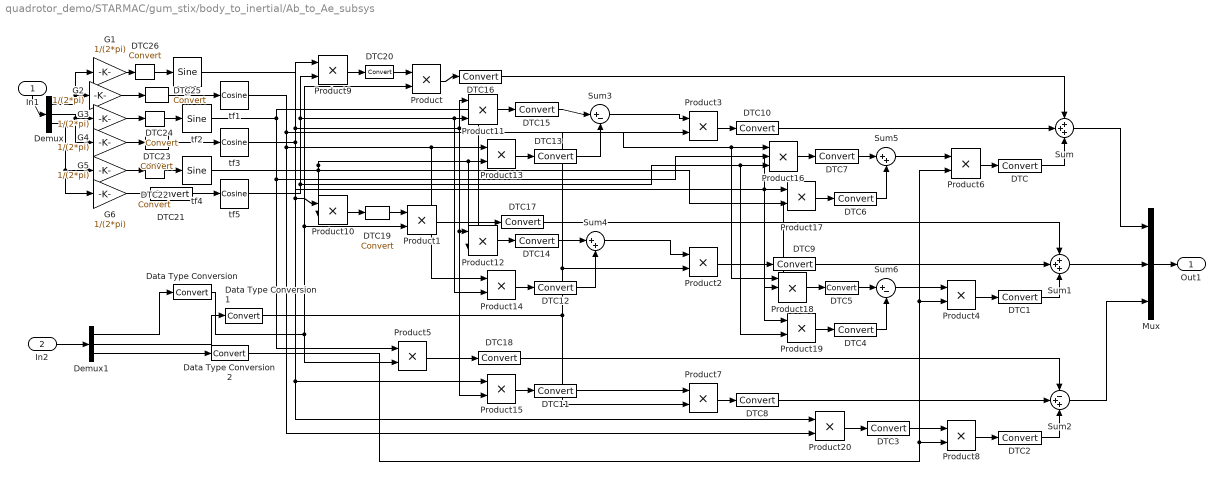
== system quadrotor_demo/STARMAC/gum_stix/body_to_inertial/Ab_to_Ae_subsys ==
  In1 : Inport
  In2 : Inport  Port=2
  DTC{,1..26} (27 alike) : DataTypeConversion
  Data Type Conversion : DataTypeConversion
  Data Type Conversion1 : DataTypeConversion
  Data Type Conversion2 : DataTypeConversion
  Demux : Demux  Outputs=3
  Demux1 : Demux  Outputs=3
  G{1..4} (4 alike) : Gain  Gain=1/(2*pi)  OutDataTypeStr=fixdt(1,32,35)
  G5 : Gain  Gain=1/(2*pi)  OutDataTypeStr=fixdt(1,32,31)
  G6 : Gain  Gain=1/(2*pi)  OutDataTypeStr=fixdt(1,32,31)
  Mux : Mux  Inputs=3
  Product{,1..3,8..9,14,20} (8 alike) : Product  OutDataTypeStr=fixdt(1,64,62)  RndMeth=Zero
  Product{5,7,10,13} (4 alike) : Product  OutDataTypeStr=fixdt(1,64,63)  RndMeth=Zero
  Product11 : Product  Inputs=3  OutDataTypeStr=fixdt(1,64,67)  RndMeth=Zero
  Product12 : Product  Inputs=3  OutDataTypeStr=fixdt(1,64,67)  RndMeth=Zero
  Product{4,6,15,17,19} (5 alike) : Product  OutDataTypeStr=fixdt(1,64,64)  RndMeth=Zero
  Product16 : Product  Inputs=3  OutDataTypeStr=fixdt(1,64,64)  RndMeth=Zero
  Product18 : Product  Inputs=3  OutDataTypeStr=fixdt(1,64,64)  RndMeth=Zero
  Sum : Sum  Inputs=+++  OutDataTypeStr=fixdt(1,32,29)
  Sum1 : Sum  Inputs=+++  OutDataTypeStr=fixdt(1,32,29)
  Sum2 : Sum  Inputs=-++  OutDataTypeStr=fixdt(1,32,29)
  Sum3 : Sum  Inputs=|+-  OutDataTypeStr=fixdt(1,32,31)
  Sum4 : Sum  Inputs=|++  OutDataTypeStr=fixdt(1,32,30)
  Sum5 : Sum  Inputs=|++  OutDataTypeStr=fixdt(1,32,32)
  Sum6 : Sum  Inputs=|+-  OutDataTypeStr=fixdt(1,32,32)
  tf : simulink/Lookup Tables/Sine  SystemSampleTime=-1  Formula=sin(2*pi*u)  NumDataPoints=(2^10)+1  OutputWordLength=32
  tf1 : simulink/Lookup Tables/Cosine  SystemSampleTime=-1  Formula=cos(2*pi*u)  NumDataPoints=(2^10)+1  OutputWordLength=32
  tf2 : simulink/Lookup Tables/Sine  SystemSampleTime=-1  Formula=sin(2*pi*u)  NumDataPoints=(2^10)+1  OutputWordLength=32
  tf3 : simulink/Lookup Tables/Cosine  SystemSampleTime=-1  Formula=cos(2*pi*u)  NumDataPoints=(2^10)+1  OutputWordLength=32
  tf4 : simulink/Lookup Tables/Sine  SystemSampleTime=-1  Formula=sin(2*pi*u)  NumDataPoints=(2^10)+1  OutputWordLength=32
  tf5 : simulink/Lookup Tables/Cosine  SystemSampleTime=-1  Formula=cos(2*pi*u)  NumDataPoints=(2^10)+1  OutputWordLength=32
  Out1 : Outport
  wires:
  Demux/1 -> G1/1, G2/1
  Demux/2 -> G3/1, G4/1
  Demux/3 -> G5/1, G6/1
  Product/1 -> DTC16/1
  Product3/1 -> DTC10/1
  Product6/1 -> DTC/1
  Product1/1 -> DTC17/1
  Product2/1 -> DTC9/1
  Product4/1 -> DTC1/1
  Product5/1 -> DTC18/1
  Product7/1 -> DTC8/1
  Product8/1 -> DTC2/1
  tf3/1 -> Product9/1, Product10/1, Product15/1, Product20/1
  tf5/1 -> Product9/2, Product11/3, Product14/2, Product16/3, Product19/2
  Product9/1 -> DTC20/1
  Demux1/1 -> Data Type Conversion/1
  tf4/1 -> Product10/2, Product13/2, Product12/3, Product17/2, Product18/3
  Product10/1 -> DTC19/1
  tf2/1 -> Product11/2, Product12/2, Product5/1, Product16/2, Product18/2
  Product11/1 -> DTC15/1
  tf/1 -> Product11/1, Product12/1, Product15/2, Product17/1, Product19/1
  tf1/1 -> Product16/1, Product18/1, Product13/1, Product14/1, Product20/2
  Product13/1 -> DTC13/1
  Sum3/1 -> Product3/1
  Demux1/2 -> Data Type Conversion1/1
  Product12/1 -> DTC14/1
  Product14/1 -> DTC12/1
  Sum4/1 -> Product2/1
  Product15/1 -> DTC11/1
  Product16/1 -> DTC7/1
  Product17/1 -> DTC6/1
  Product18/1 -> DTC5/1
  Product19/1 -> DTC4/1
  Sum5/1 -> Product6/1
  Sum6/1 -> Product4/1
  Product20/1 -> DTC3/1
  Demux1/3 -> Data Type Conversion2/1
  Sum/1 -> Mux/1
  Sum1/1 -> Mux/2
  Sum2/1 -> Mux/3
  In1/1 -> Demux/1
  In2/1 -> Demux1/1
  Mux/1 -> Out1/1
  G1/1 -> DTC26/1
  G2/1 -> DTC25/1
  G3/1 -> DTC24/1
  G4/1 -> DTC23/1
  G5/1 -> DTC22/1
  G6/1 -> DTC21/1
  DTC/1 -> Sum/3
  DTC1/1 -> Sum1/3
  DTC2/1 -> Sum2/3
  DTC3/1 -> Product8/1
  DTC4/1 -> Sum6/2
  DTC5/1 -> Sum6/1
  DTC6/1 -> Sum5/2
  DTC7/1 -> Sum5/1
  DTC8/1 -> Sum2/2
  DTC9/1 -> Sum1/2
  DTC10/1 -> Sum/2
  DTC11/1 -> Product7/1
  DTC12/1 -> Sum4/2
  DTC13/1 -> Sum3/2
  DTC14/1 -> Sum4/1
  DTC15/1 -> Sum3/1
  DTC16/1 -> Sum/1
  DTC17/1 -> Sum1/1
  DTC18/1 -> Sum2/1
  DTC19/1 -> Product1/1
  DTC20/1 -> Product/1
  DTC21/1 -> tf5/1
  DTC22/1 -> tf4/1
  DTC23/1 -> tf3/1
  DTC24/1 -> tf2/1
  DTC25/1 -> tf1/1
  DTC26/1 -> tf/1
  Data Type Conversion/1 -> Product/2, Product1/2, Product5/2
  Data Type Conversion1/1 -> Product3/2, Product2/2, Product7/2
  Data Type Conversion2/1 -> Product8/2, Product4/2, Product6/2

== system quadrotor_demo/STARMAC/gum_stix/body_to_inertial/inertial_vel_and pos_est ==
  Ab : Inport
  DT_integrator : Subsystem
  DT_integrator1 : Subsystem
  Vb : Outport
  Xb : Outport  Port=2
  wires:
  DT_integrator1/1(Xb) -> Xb/1
  Ab/1 -> DT_integrator/1(Ab)
  DT_integrator/1(Vb) -> Vb/1, DT_integrator1/1(Vb)

== system quadrotor_demo/STARMAC/gum_stix/inertial_pos_controller/input_filter ==
  yaw_set : Inport
  DTC : DataTypeConversion
  Discrete Transfer Fcn : DiscreteTransferFcn  Numerator=Hz.num{1}  Denominator=Hz.den{1}  SampleTime=-1
  yaw_r : Outport
  wires:
  yaw_set/1 -> Discrete Transfer Fcn/1
  Discrete Transfer Fcn/1 -> DTC/1
  DTC/1 -> yaw_r/1

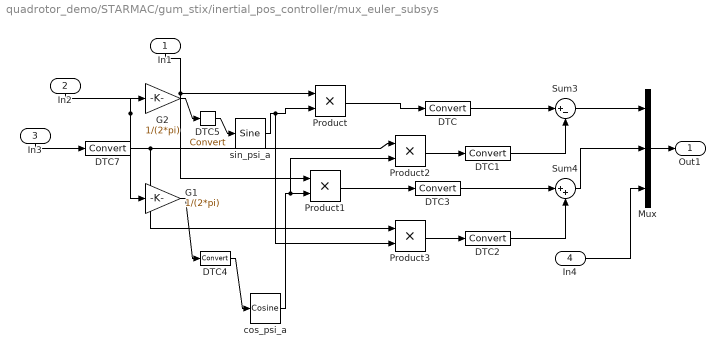
== system quadrotor_demo/STARMAC/gum_stix/inertial_pos_controller/mux_euler_subsys ==
  In1 : Inport
  In2 : Inport  Port=2
  In3 : Inport  Port=3
  In4 : Inport  Port=4
  DTC{,1..5,7} (7 alike) : DataTypeConversion
  G1 : Gain  Gain=1/(2*pi)  OutDataTypeStr=fixdt(1,32,31)
  G2 : Gain  Gain=1/(2*pi)  OutDataTypeStr=fixdt(1,32,31)
  Mux : Mux  Inputs=3
  Product{,1..3} (4 alike) : Product  OutDataTypeStr=fixdt(1,64,62)  RndMeth=Zero
  Sum3 : Sum  Inputs=|+-  OutDataTypeStr=fixdt(1,32,29)
  Sum4 : Sum  Inputs=|++  OutDataTypeStr=fixdt(1,32,29)
  cos_psi_a : simulink/Lookup Tables/Cosine  SystemSampleTime=-1  Formula=cos(2*pi*u)  NumDataPoints=(2^10)+1  OutputWordLength=32
  sin_psi_a : simulink/Lookup Tables/Sine  SystemSampleTime=-1  Formula=sin(2*pi*u)  NumDataPoints=(2^10)+1  OutputWordLength=32
  Out1 : Outport
  wires:
  sin_psi_a/1 -> Product/2, Product3/2
  Product/1 -> DTC/1
  cos_psi_a/1 -> Product2/2, Product1/2
  Product2/1 -> DTC1/1
  Product1/1 -> DTC3/1
  Product3/1 -> DTC2/1
  Sum3/1 -> Mux/1
  Sum4/1 -> Mux/2
  In1/1 -> Product1/1, Product/1
  In2/1 -> G1/1, G2/1
  In3/1 -> DTC7/1
  Mux/1 -> Out1/1
  In4/1 -> Mux/3
  G1/1 -> DTC4/1
  G2/1 -> DTC5/1
  DTC/1 -> Sum3/1
  DTC1/1 -> Sum3/2
  DTC2/1 -> Sum4/2
  DTC3/1 -> Sum4/1
  DTC4/1 -> cos_psi_a/1
  DTC5/1 -> sin_psi_a/1
  DTC7/1 -> Product2/1, Product3/1

== system quadrotor_demo/STARMAC/gum_stix/inertial_pos_controller/vel_est ==
  Xe_set : Inport
  DTC1 : DataTypeConversion
  DTC2 : DataTypeConversion
  DTC22 : DataTypeConversion
  Demux : Demux  Outputs=3
  Discrete Transfer Fcn : DiscreteTransferFcn  Numerator=Hz.num{1}  Denominator=Hz.den{1}  SampleTime=-1
  Discrete Transfer Fcn1 : DiscreteTransferFcn  Numerator=Hz.num{1}  Denominator=Hz.den{1}  SampleTime=-1
  Discrete Transfer Fcn2 : DiscreteTransferFcn  Numerator=Hz.num{1}  Denominator=Hz.den{1}  SampleTime=-1
  Mux : Mux  Inputs=3
  Ve_set : Outport
  wires:
  Xe_set/1 -> Demux/1  "x"
  Demux/1 -> Discrete Transfer Fcn/1
  Demux/2 -> Discrete Transfer Fcn1/1
  Demux/3 -> Discrete Transfer Fcn2/1
  Mux/1 -> Ve_set/1
  Discrete Transfer Fcn/1 -> DTC2/1
  Discrete Transfer Fcn1/1 -> DTC1/1
  Discrete Transfer Fcn2/1 -> DTC22/1
  DTC22/1 -> Mux/3
  DTC1/1 -> Mux/2
  DTC2/1 -> Mux/1

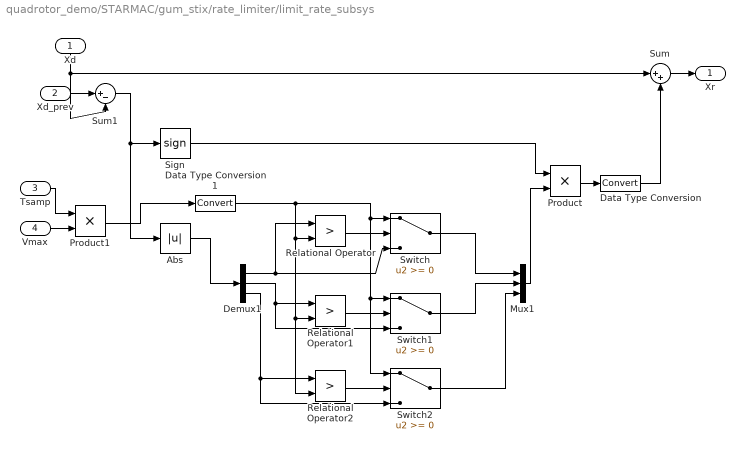
== system quadrotor_demo/STARMAC/gum_stix/rate_limiter/limit_rate_subsys ==
  Xd : Inport
  Xd_prev : Inport  Port=2
  Tsamp : Inport  Port=3
  Vmax : Inport  Port=4
  Abs : Abs
  Data Type Conversion : DataTypeConversion
  Data Type Conversion1 : DataTypeConversion
  Demux1 : Demux  Outputs=3
  Mux1 : Mux  Inputs=3
  Product : Product  RndMeth=Zero
  Product1 : Product  RndMeth=Zero
  Relational Operator : RelationalOperator  Operator=>  OutDataTypeStr=boolean
  Relational Operator1 : RelationalOperator  Operator=>  OutDataTypeStr=boolean
  Relational Operator2 : RelationalOperator  Operator=>  OutDataTypeStr=boolean
  Sign : Signum
  Sum : Sum  Inputs=|++
  Sum1 : Sum  Inputs=|+-
  Switch : Switch
  Switch1 : Switch
  Switch2 : Switch
  Xr : Outport
  wires:
  Xd/1 -> Sum1/2, Sum/1
  Sum1/1 -> Sign/1, Abs/1
  Sign/1 -> Product/1
  Relational Operator/1 -> Switch/2
  Demux1/1 -> Switch/3, Relational Operator/1
  Switch/1 -> Mux1/1
  Abs/1 -> Demux1/1
  Product1/1 -> Data Type Conversion1/1
  Relational Operator1/1 -> Switch1/2
  Demux1/2 -> Relational Operator1/1, Switch1/3
  Switch1/1 -> Mux1/2
  Relational Operator2/1 -> Switch2/2
  Demux1/3 -> Relational Operator2/1, Switch2/3
  Switch2/1 -> Mux1/3
  Mux1/1 -> Product/2
  Product/1 -> Data Type Conversion/1
  Sum/1 -> Xr/1
  Xd_prev/1 -> Sum1/1
  Tsamp/1 -> Product1/1
  Vmax/1 -> Product1/2
  Data Type Conversion/1 -> Sum/2
  Data Type Conversion1/1 -> Relational Operator/2, Relational Operator1/2, Relational Operator2/2, Switch/1, Switch1/1, Switch2/1

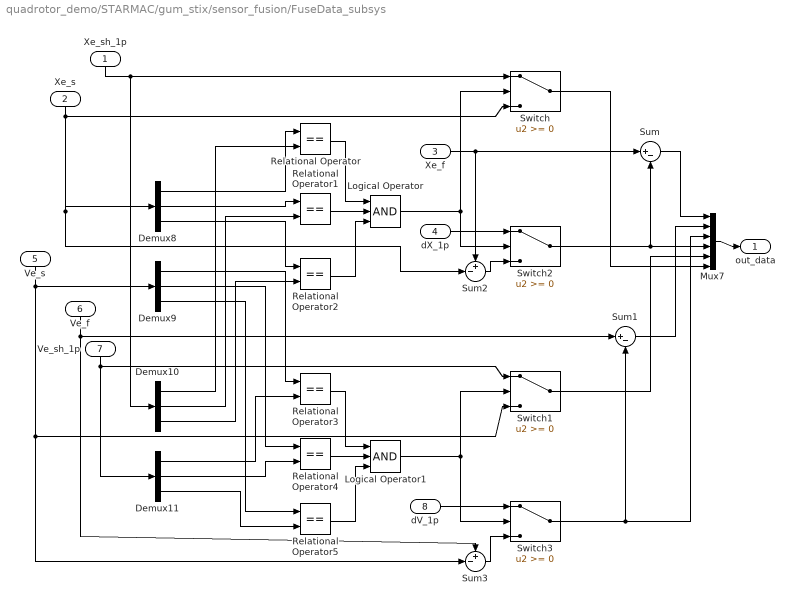
== system quadrotor_demo/STARMAC/gum_stix/sensor_fusion/FuseData_subsys ==
  Xe_sh_1p : Inport
  Xe_s : Inport  Port=2
  Xe_f : Inport  Port=3
  dX_1p : Inport  Port=4
  Ve_s : Inport  Port=5
  Ve_f : Inport  Port=6
  Ve_sh_1p : Inport  Port=7
  dV_1p : Inport  Port=8
  Demux{8..11} (4 alike) : Demux  Outputs=3
  Logical Operator : Logic  Inputs=3  AllPortsSameDT=off  OutDataTypeStr=boolean
  Logical Operator1 : Logic  Inputs=3  AllPortsSameDT=off  OutDataTypeStr=boolean
  Mux7 : Mux  Inputs=6
  Relational Operator{,1..5} (6 alike) : RelationalOperator  Operator===  OutDataTypeStr=boolean
  Sum : Sum  Inputs=|+-  OutDataTypeStr=fixdt(1,32,19)
  Sum1 : Sum  Inputs=|+-  OutDataTypeStr=fixdt(1,32,19)
  Sum2 : Sum  Inputs=+-|  OutDataTypeStr=fixdt(1,32,19)
  Sum3 : Sum  Inputs=+-|  OutDataTypeStr=fixdt(1,32,24)
  Switch{,1..3} (4 alike) : Switch  OutDataTypeStr=fixdt(1,32,19)
  out_data : Outport
  wires:
  Relational Operator/1 -> Logical Operator/1
  Relational Operator1/1 -> Logical Operator/2
  Relational Operator2/1 -> Logical Operator/3
  Logical Operator/1 -> Switch/2, Switch2/2
  Relational Operator3/1 -> Logical Operator1/1
  Relational Operator4/1 -> Logical Operator1/2
  Relational Operator5/1 -> Logical Operator1/3
  Logical Operator1/1 -> Switch1/2, Switch3/2
  Switch2/1 -> Mux7/4, Sum/2
  Switch/1 -> Mux7/6
  Switch1/1 -> Mux7/5
  Switch3/1 -> Mux7/3, Sum1/2
  Sum/1 -> Mux7/1
  Sum1/1 -> Mux7/2
  Demux8/1 -> Relational Operator/1
  Demux10/1 -> Relational Operator/2
  Demux8/2 -> Relational Operator1/1
  Demux10/2 -> Relational Operator1/2
  Demux8/3 -> Relational Operator2/1
  Demux10/3 -> Relational Operator2/2
  Demux9/1 -> Relational Operator3/1
  Demux9/2 -> Relational Operator4/1
  Demux9/3 -> Relational Operator5/1
  Demux11/1 -> Relational Operator3/2
  Demux11/2 -> Relational Operator4/2
  Demux11/3 -> Relational Operator5/2
  Sum2/1 -> Switch2/3
  Sum3/1 -> Switch3/3
  Xe_sh_1p/1 -> Switch/1, Demux10/1
  Xe_s/1 -> Switch/3, Demux8/1, Sum2/2
  Xe_f/1 -> Sum/1, Sum2/1
  dX_1p/1 -> Switch2/1
  Ve_s/1 -> Switch1/3, Sum3/2, Demux9/1
  Ve_f/1 -> Sum1/1, Sum3/1
  Ve_sh_1p/1 -> Demux11/1, Switch1/1
  dV_1p/1 -> Switch3/1
  Mux7/1 -> out_data/1

== system quadrotor_demo/STARMAC/robo_stix/inner_loop/euler_controller ==
  euler_set : Inport  PortDimensions=[3]
  euler : Inport  Port=2  PortDimensions=[3]
  omega : Inport  Port=3  PortDimensions=[3]
  Data Type Conversion : DataTypeConversion  OutDataTypeStr=fixdt(1,32,34)
  Data Type Conversion1 : DataTypeConversion
  K_euler : Gain  Gain=single(K_e)
  K_omega : Gain  Gain=single(K_o)
  Sum : Sum  Inputs=|+-
  Sum1 : Sum  Inputs=|+-
  torque_limit : Saturate  UpperLimit=9.8*.3048*ones(3,1)  LowerLimit=-9.8*.3048*ones(3,1)  OutDataTypeStr=Inherit: Inherit via back propagation
  u_torque : Outport
  wires:
  Sum/1 -> K_omega/1
  euler_set/1 -> Sum1/1  "euler_set"
  Sum1/1 -> K_euler/1
  euler/1 -> Sum1/2  "euler"
  K_euler/1 -> Data Type Conversion1/1  "u_omega"
  torque_limit/1 -> u_torque/1
  K_omega/1 -> Data Type Conversion/1
  omega/1 -> Sum/2  "omega"
  Data Type Conversion/1 -> torque_limit/1
  Data Type Conversion1/1 -> Sum/1

== system quadrotor_demo/STARMAC/robo_stix/inner_loop/lead_motor ==
  thrust_in : Inport  PortDimensions=[4]
  Data Type Conversion{,1..3} (4 alike) : DataTypeConversion
  Demux : Demux
  Discrete Transfer Fcn{,1..3} (4 alike) : DiscreteTransferFcn  Numerator=Hzn1  Denominator=Hzd1  SampleTime=-1
  Mux : Mux
  thrust_out : Outport
  wires:
  thrust_in/1 -> Demux/1  "x"
  Demux/1 -> Discrete Transfer Fcn/1
  Demux/2 -> Discrete Transfer Fcn1/1
  Demux/3 -> Discrete Transfer Fcn2/1
  Mux/1 -> thrust_out/1
  Discrete Transfer Fcn/1 -> Data Type Conversion3/1
  Discrete Transfer Fcn1/1 -> Data Type Conversion2/1
  Discrete Transfer Fcn2/1 -> Data Type Conversion1/1
  Demux/4 -> Discrete Transfer Fcn3/1
  Discrete Transfer Fcn3/1 -> Data Type Conversion/1
  Data Type Conversion/1 -> Mux/4
  Data Type Conversion1/1 -> Mux/3
  Data Type Conversion2/1 -> Mux/2
  Data Type Conversion3/1 -> Mux/1

== system quadrotor_demo/STARMAC/robo_stix/inner_loop/u_T_u_torque_motor_thrust ==
  u_torque : Inport  PortDimensions=[3]
  u_T : Inport  Port=2  PortDimensions=[1]
  Data Type Conversion : DataTypeConversion  OutDataTypeStr=fixdt(1,32,31)
  Mi : Gain  Gain=Mi  Multiplication=Matrix(K*u)
  Mux : Mux  Inputs=2
  u_torque_u_T_mux : Stateflow chart  TreatAsAtomicUnit=on
  cont_motor_thrust : Outport
  wires:
  u_torque/1 -> Mux/1
  u_T/1 -> Mux/2
  Mi/1 -> Data Type Conversion/1
  Mux/1 -> Mi/1
  Data Type Conversion/1 -> cont_motor_thrust/1

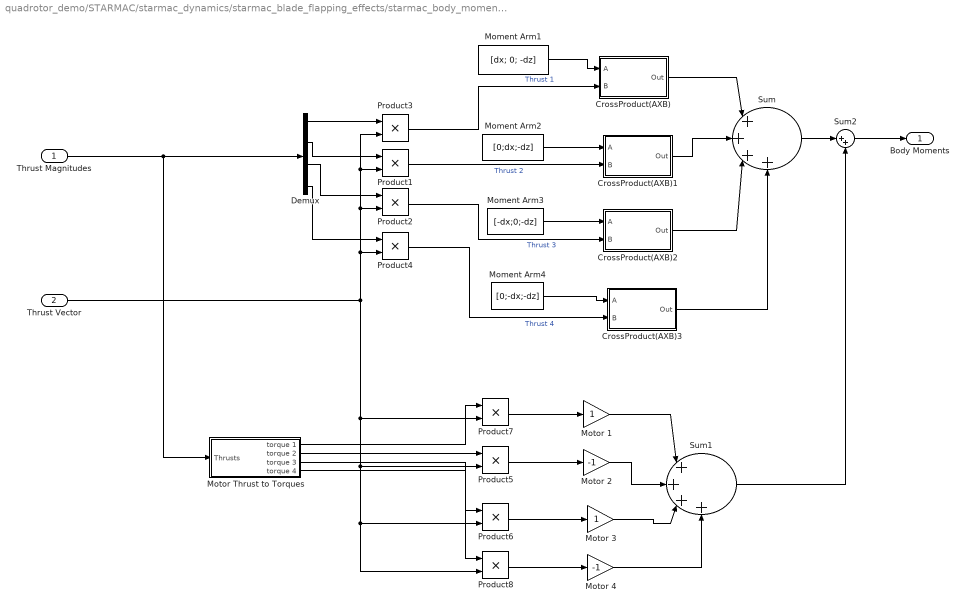
== system quadrotor_demo/STARMAC/starmac_dynamics/starmac_blade_flapping_effects/starmac_body_moments ==
  Thrust Magnitudes : Inport
  Thrust Vector : Inport  Port=2
  CrossProduct(AXB) : Subsystem
  CrossProduct(AXB)1 : Subsystem
  CrossProduct(AXB)2 : Subsystem
  CrossProduct(AXB)3 : Subsystem
  Demux : Demux
  Moment Arm1 : Constant  Value=[dx; 0; -dz]
  Moment Arm2 : Constant  Value=[0;dx;-dz]
  Moment Arm3 : Constant  Value=[-dx;0;-dz]
  Moment Arm4 : Constant  Value=[0;-dx;-dz]
  Motor 1 : Gain  OutDataTypeStr=single
  Motor 2 : Gain  Gain=-1  OutDataTypeStr=single
  Motor 3 : Gain  OutDataTypeStr=single
  Motor 4 : Gain  Gain=-1  OutDataTypeStr=single
  Motor Thrust to Torques : Subsystem
  Product{1..8} (8 alike) : Product  RndMeth=Zero
  Sum : Sum  Inputs=|++++
  Sum1 : Sum  Inputs=|++++
  Sum2 : Sum  Inputs=|++
  Body Moments : Outport
  wires:
  CrossProduct(AXB)1/1(Out) -> Sum/2
  Motor Thrust to Torques/4(torque 4) -> Product8/1
  Motor Thrust to Torques/3(torque 3) -> Product6/1
  Motor Thrust to Torques/2(torque 2) -> Product5/1
  Motor Thrust to Torques/1(torque 1) -> Product7/1
  Product8/1 -> Motor 4/1
  Product6/1 -> Motor 3/1
  Product5/1 -> Motor 2/1
  Product7/1 -> Motor 1/1
  Sum2/1 -> Body Moments/1
  Sum1/1 -> Sum2/2
  Sum/1 -> Sum2/1
  Motor 4/1 -> Sum1/4
  Motor 3/1 -> Sum1/3
  Motor 2/1 -> Sum1/2
  Motor 1/1 -> Sum1/1
  CrossProduct(AXB)3/1(Out) -> Sum/4
  CrossProduct(AXB)2/1(Out) -> Sum/3
  CrossProduct(AXB)/1(Out) -> Sum/1
  Product4/1 -> CrossProduct(AXB)3/2(B)  "Thrust 4"
  Moment Arm4/1 -> CrossProduct(AXB)3/1(A)
  Product2/1 -> CrossProduct(AXB)2/2(B)  "Thrust 3"
  Moment Arm3/1 -> CrossProduct(AXB)2/1(A)
  Product1/1 -> CrossProduct(AXB)1/2(B)  "Thrust 2"
  Moment Arm2/1 -> CrossProduct(AXB)1/1(A)
  Product3/1 -> CrossProduct(AXB)/2(B)  "Thrust 1"
  Moment Arm1/1 -> CrossProduct(AXB)/1(A)
  Thrust Vector/1 -> Product8/2, Product6/2, Product5/2, Product7/2, Product4/2, Product2/2, Product1/2, Product3/2
  Demux/4 -> Product4/1
  Demux/3 -> Product2/1
  Demux/2 -> Product1/1
  Demux/1 -> Product3/1
  Thrust Magnitudes/1 -> Motor Thrust to Torques/1(Thrusts), Demux/1

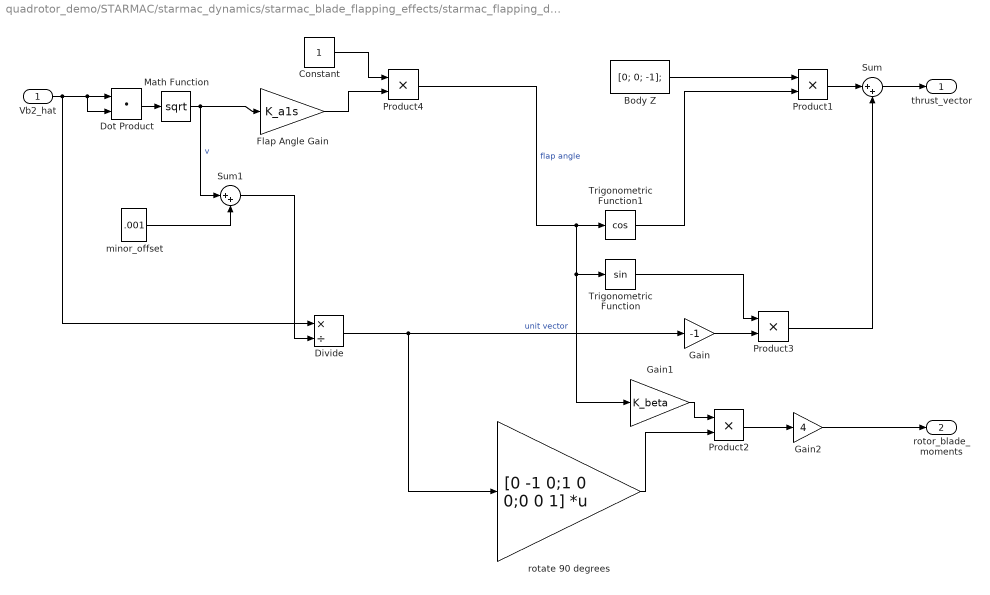
== system quadrotor_demo/STARMAC/starmac_dynamics/starmac_blade_flapping_effects/starmac_flapping_dynamics ==
  Vb2_hat : Inport
  "Body Z " : Constant  Value=[0; 0; -1];
  Constant : Constant
  Divide : Product  Inputs=*/
  Dot Product : DotProduct  InputSameDT=on  OutDataTypeStr=Inherit: Inherit via internal rule
  Flap Angle Gain : Gain  Gain=K_a1s  OutDataTypeStr=single
  Gain : Gain  Gain=-1  OutDataTypeStr=single
  Gain1 : Gain  Gain=K_beta  OutDataTypeStr=single
  Gain2 : Gain  Gain=4  OutDataTypeStr=single
  Math Function : Math  Operator=sqrt  SaturateOnIntegerOverflow=on
  Product{1..4} (4 alike) : Product  RndMeth=Zero
  Sum : Sum  Inputs=|++
  Sum1 : Sum  Inputs=|++
  Trigonometric Function : Trigonometry
  Trigonometric Function1 : Trigonometry  Operator=cos
  minor_offset : Constant  Value=.001
  rotate 90 degrees : Gain  Gain=[0 -1 0;1 0 0;0 0 1]  Multiplication=Matrix(K*u)  OutDataTypeStr=single
  thrust_vector : Outport
  rotor_blade_moments : Outport  Port=2
  wires:
  minor_offset/1 -> Sum1/2
  Sum1/1 -> Divide/2
  Divide/1 -> rotate 90 degrees/1, Gain/1  "unit vector"
  Product4/1 -> Trigonometric Function1/1, Trigonometric Function/1, Gain1/1  "flap angle"
  Vb2_hat/1 -> Divide/1, Dot Product/1, Dot Product/2
  Dot Product/1 -> Math Function/1
  Math Function/1 -> Sum1/1, Flap Angle Gain/1  "v"
  Trigonometric Function1/1 -> Product1/2
  Trigonometric Function/1 -> Product3/1
  Product3/1 -> Sum/2
  Gain/1 -> Product3/2
  Product1/1 -> Sum/1
  "Body Z "/1 -> Product1/1
  Sum/1 -> thrust_vector/1
  Gain2/1 -> rotor_blade_moments/1
  Product2/1 -> Gain2/1
  rotate 90 degrees/1 -> Product2/2
  Gain1/1 -> Product2/1
  Flap Angle Gain/1 -> Product4/2
  Constant/1 -> Product4/1

== system quadrotor_demo/STARMAC/starmac_dynamics/starmac_blade_flapping_effects/starmac_vertical_effect_dynamics ==
  motor_thrusts : Inport
  v_body_relative : Inport  Port=2
  Demux : Demux
  Mux : Mux
  starmac_motor_vertical_effect_dynamics{,1..3} (4 alike) : aero_sim_lib/starmac_motor_vertical_effect_dynamics  SystemSampleTime=-1  tau_motor=tau_motor  R=R  Alpha=Alpha  Vinf=Vinf  Vh=Vh  ToverTh=ToverTh
  thrust_multiplier : Outport
  wires:
  motor_thrusts/1 -> Demux/1
  Mux/1 -> thrust_multiplier/1
  Demux/1 -> starmac_motor_vertical_effect_dynamics/1
  Demux/2 -> starmac_motor_vertical_effect_dynamics1/1
  Demux/3 -> starmac_motor_vertical_effect_dynamics2/1
  Demux/4 -> starmac_motor_vertical_effect_dynamics3/1
  starmac_motor_vertical_effect_dynamics/1 -> Mux/1
  starmac_motor_vertical_effect_dynamics1/1 -> Mux/2
  starmac_motor_vertical_effect_dynamics2/1 -> Mux/3
  starmac_motor_vertical_effect_dynamics3/1 -> Mux/4
  v_body_relative/1 -> starmac_motor_vertical_effect_dynamics2/2, starmac_motor_vertical_effect_dynamics3/2, starmac_motor_vertical_effect_dynamics1/2, starmac_motor_vertical_effect_dynamics/2

== system quadrotor_demo/STARMAC/gum_stix/body_to_inertial/inertial_vel_and pos_est/DT_integrator ==
  Ab : Inport
  DTC : DataTypeConversion  OutDataTypeStr=fixdt(1,32,33)
  Sum : Sum  Inputs=++|
  Sum1 : Sum  Inputs=|++
  negate : Gain  Gain=.5*Ts
  u_delay : UnitDelay  SampleTime=-1
  u_delay1 : UnitDelay  SampleTime=-1
  Vb : Outport
  wires:
  Ab/1 -> u_delay/1, Sum/2
  u_delay/1 -> Sum/1
  Sum/1 -> negate/1
  negate/1 -> DTC/1
  Sum1/1 -> u_delay1/1, Vb/1
  u_delay1/1 -> Sum1/2
  DTC/1 -> Sum1/1

== system quadrotor_demo/STARMAC/gum_stix/body_to_inertial/inertial_vel_and pos_est/DT_integrator1 ==
  Vb : Inport
  DTC : DataTypeConversion  OutDataTypeStr=fixdt(1,32,35)
  Sum : Sum  Inputs=++|
  Sum1 : Sum  Inputs=|++
  negate : Gain  Gain=.5*Ts
  u_delay : UnitDelay  SampleTime=-1
  u_delay1 : UnitDelay  SampleTime=-1
  Xb : Outport  PortDimensions=[3]
  wires:
  u_delay1/1 -> Sum1/2
  Sum1/1 -> Xb/1, u_delay1/1
  negate/1 -> DTC/1
  Sum/1 -> negate/1
  u_delay/1 -> Sum/1
  Vb/1 -> Sum/2, u_delay/1
  DTC/1 -> Sum1/1

== system quadrotor_demo/STARMAC/starmac_dynamics/starmac_blade_flapping_effects/starmac_body_moments/CrossProduct(AXB) ==
  A : Inport
  B : Inport  Port=2
  Fcn : Fcn  Expr=u[2]*u[6]-u[3]*u[5]
  Fcn1 : Fcn  Expr=u[3]*u[4]-u[1]*u[6]
  Fcn2 : Fcn  Expr=u[1]*u[5]-u[2]*u[4]
  Mux : Mux  Inputs=2
  Mux1 : Mux  Inputs=3
  Out : Outport
  wires:
  Mux1/1 -> Out/1
  Fcn2/1 -> Mux1/3
  Fcn1/1 -> Mux1/2
  Fcn/1 -> Mux1/1
  Mux/1 -> Fcn2/1, Fcn1/1, Fcn/1
  B/1 -> Mux/2
  A/1 -> Mux/1

== system quadrotor_demo/STARMAC/starmac_dynamics/starmac_blade_flapping_effects/starmac_body_moments/CrossProduct(AXB)1 ==
  A : Inport
  B : Inport  Port=2
  Fcn : Fcn  Expr=u[2]*u[6]-u[3]*u[5]
  Fcn1 : Fcn  Expr=u[3]*u[4]-u[1]*u[6]
  Fcn2 : Fcn  Expr=u[1]*u[5]-u[2]*u[4]
  Mux : Mux  Inputs=2
  Mux1 : Mux  Inputs=3
  Out : Outport
  wires:
  A/1 -> Mux/1
  B/1 -> Mux/2
  Mux/1 -> Fcn/1, Fcn1/1, Fcn2/1
  Fcn/1 -> Mux1/1
  Fcn1/1 -> Mux1/2
  Fcn2/1 -> Mux1/3
  Mux1/1 -> Out/1

== system quadrotor_demo/STARMAC/starmac_dynamics/starmac_blade_flapping_effects/starmac_body_moments/CrossProduct(AXB)2 ==
  A : Inport
  B : Inport  Port=2
  Fcn : Fcn  Expr=u[2]*u[6]-u[3]*u[5]
  Fcn1 : Fcn  Expr=u[3]*u[4]-u[1]*u[6]
  Fcn2 : Fcn  Expr=u[1]*u[5]-u[2]*u[4]
  Mux : Mux  Inputs=2
  Mux1 : Mux  Inputs=3
  Out : Outport
  wires:
  Mux1/1 -> Out/1
  Fcn2/1 -> Mux1/3
  Fcn1/1 -> Mux1/2
  Fcn/1 -> Mux1/1
  Mux/1 -> Fcn2/1, Fcn1/1, Fcn/1
  B/1 -> Mux/2
  A/1 -> Mux/1

== system quadrotor_demo/STARMAC/starmac_dynamics/starmac_blade_flapping_effects/starmac_body_moments/CrossProduct(AXB)3 ==
  A : Inport
  B : Inport  Port=2
  Fcn : Fcn  Expr=u[2]*u[6]-u[3]*u[5]
  Fcn1 : Fcn  Expr=u[3]*u[4]-u[1]*u[6]
  Fcn2 : Fcn  Expr=u[1]*u[5]-u[2]*u[4]
  Mux : Mux  Inputs=2
  Mux1 : Mux  Inputs=3
  Out : Outport
  wires:
  A/1 -> Mux/1
  B/1 -> Mux/2
  Mux/1 -> Fcn/1, Fcn1/1, Fcn2/1
  Fcn/1 -> Mux1/1
  Fcn1/1 -> Mux1/2
  Fcn2/1 -> Mux1/3
  Mux1/1 -> Out/1
